simulink subsystem "propulsion"  (R2024b)
settings: Solver=VariableStepAuto  StartTime=0.0  StopTime=10.0  RelTol=1e-3
undefined symbols (not defined in the file or in its folder): aexit, prop_cg_t, prop_cg_v, prop_mass_t, prop_mass_v, prop_moipitch_t, prop_moipitch_v, prop_moiroll_t, prop_moiroll_v, prop_thrust_t, prop_thrust_v
settings Model: Creator=yagiz  LastModifiedBy=yagiz

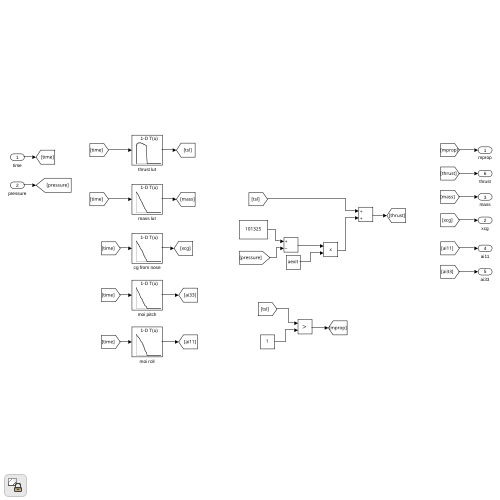
[thumbnail: Simulink's stored preview of the top-level diagram]
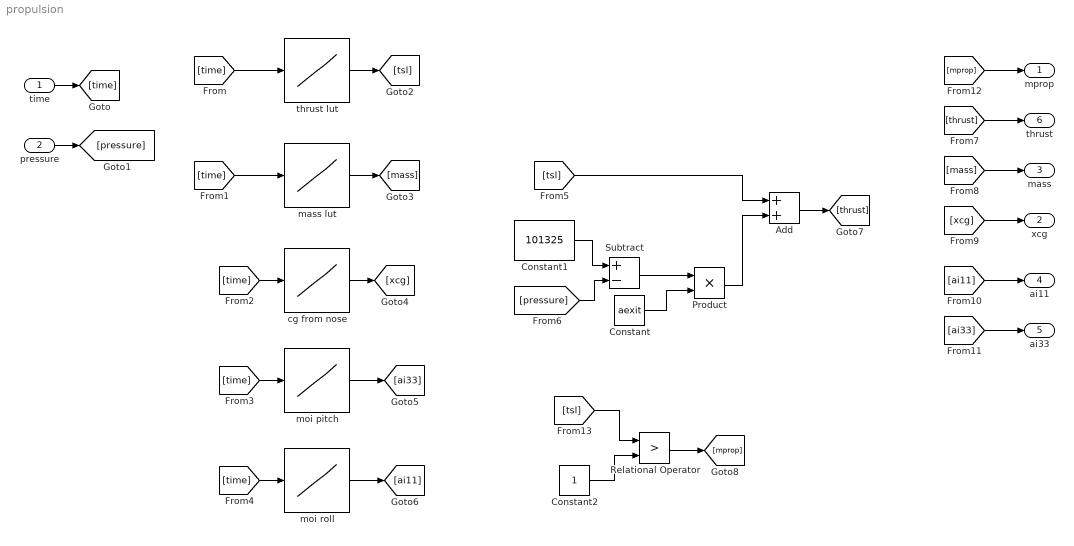
== system propulsion ==
  time : Inport
  pressure : Inport  Port=2
  Add : Sum
  Constant : Constant  Value=aexit
  Constant1 : Constant  Value=101325
  Constant2 : Constant
  Product : Product
  Relational Operator : RelationalOperator  Operator=>  OutDataTypeStr=boolean  RndMeth=Simplest  InputSameDT=off
  Subtract : Sum  Inputs=+-
  cg from nose : Lookup_n-D  NumberOfTableDimensions=1  BreakpointsForDimension1=prop_cg_t  Table=prop_cg_v  ExtrapMethod=Clip  UseLastTableValue=on  InternalRulePriority=Speed  RndMeth=Simplest
  mass lut : Lookup_n-D  NumberOfTableDimensions=1  BreakpointsForDimension1=prop_mass_t  Table=prop_mass_v  ExtrapMethod=Clip  UseLastTableValue=on  InternalRulePriority=Speed  RndMeth=Simplest
  moi pitch : Lookup_n-D  NumberOfTableDimensions=1  BreakpointsForDimension1=prop_moipitch_t  Table=prop_moipitch_v  ExtrapMethod=Clip  UseLastTableValue=on  InternalRulePriority=Speed  RndMeth=Simplest
  moi roll : Lookup_n-D  NumberOfTableDimensions=1  BreakpointsForDimension1=prop_moiroll_t  Table=prop_moiroll_v  ExtrapMethod=Clip  UseLastTableValue=on  InternalRulePriority=Speed  RndMeth=Simplest
  thrust lut : Lookup_n-D  NumberOfTableDimensions=1  BreakpointsForDimension1=prop_thrust_t  Table=prop_thrust_v  ExtrapMethod=Clip  UseLastTableValue=on  InternalRulePriority=Speed  RndMeth=Simplest
  mprop : Outport
  xcg : Outport  Port=2
  mass : Outport  Port=3
  ai11 : Outport  Port=4
  ai33 : Outport  Port=5
  thrust : Outport  Port=6
  wires:
  time/1 -> [time]
  pressure/1 -> [pressure]
  [time] -> thrust lut/1
  [time] -> mass lut/1
  [time] -> cg from nose/1
  [time] -> moi pitch/1
  [time] -> moi roll/1
  thrust lut/1 -> [tsl]
  mass lut/1 -> [mass]
  cg from nose/1 -> [xcg]
  moi pitch/1 -> [ai33]
  moi roll/1 -> [ai11]
  [tsl] -> Add/1
  Constant1/1 -> Subtract/1
  [pressure] -> Subtract/2
  Subtract/1 -> Product/1
  Constant/1 -> Product/2
  Product/1 -> Add/2
  Add/1 -> [thrust]
  [thrust] -> thrust/1
  [mass] -> mass/1
  [xcg] -> xcg/1
  [ai33] -> ai33/1
  [ai11] -> ai11/1
  Relational Operator/1 -> [mprop]
  [tsl] -> Relational Operator/1
  Constant2/1 -> Relational Operator/2
  [mprop] -> mprop/1
